simulink model "dynamics_updated"  (R2025b)
settings: Solver=VariableStepAuto  StartTime=0.0  StopTime=10.0  RelTol=1e-3
settings Model: Creator=koryh  LastModifiedBy=koryh

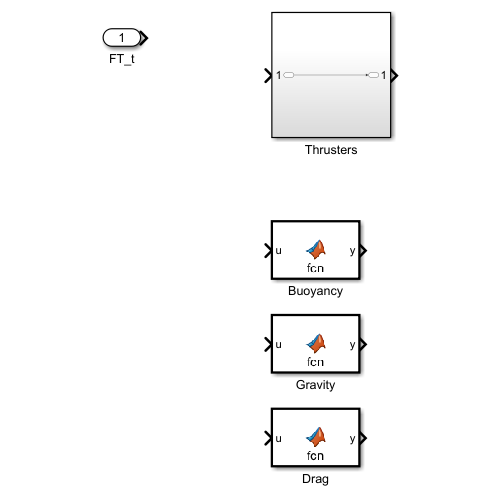
[thumbnail: Simulink's stored preview of the top-level diagram]
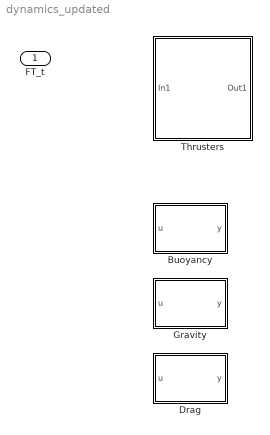
== system dynamics_updated ==
  FT_t : Inport
  Buoyancy : MATLAB Function  TreatAsAtomicUnit=on
  Drag : MATLAB Function  TreatAsAtomicUnit=on
  Gravity : MATLAB Function  TreatAsAtomicUnit=on
  Thrusters : Subsystem

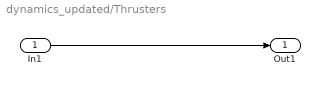
== system dynamics_updated/Thrusters ==
  In1 : Inport
  Out1 : Outport
  wires:
  In1/1 -> Out1/1

== matlab function dynamics_updated/Buoyancy ==
  data: u input; y output
function y = fcn(u)

y = u;

== matlab function dynamics_updated/Drag ==
  data: u input; y output
function y = fcn(u)

y = u;

== matlab function dynamics_updated/Gravity ==
  data: u input; y output
function y = fcn(u)

y = u;
